simulink model "integrator_ext_IC_test"  (Simulink 8.7)
settings: Solver=ode45  StartTime=0.0  StopTime=10.0  RelTol=1e-3
undefined symbols (not defined in the file or in its folder): DiscIntNeverNeededParam
settings Model: Creator=arnaud  LastModifiedBy=hamza
settings DataIOCC: SaveFormat=Structure  SignalLoggingSaveFormat=ModelDataLogs
settings OptimizationCC: ExpressionDepthLimit=2147483647
settings DebuggingCC: SolverPrmCheckMsg=warning  FcnCallInpInsideContextMsg=UseLocalSettings  StateNameClashWarn=warning
settings GRTTargetCC: CombineOutputUpdateFcns=off  GRTInterface=on
settings ConfigComp: CovSFcnEnable=off

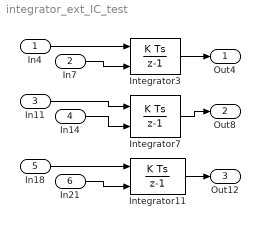
== system integrator_ext_IC_test ==
  In4 : Inport  OutDataTypeStr=double
  In7 : Inport  Port=2  OutDataTypeStr=double
  In11 : Inport  Port=3  OutDataTypeStr=int32
  In14 : Inport  Port=4  OutDataTypeStr=int32
  In18 : Inport  Port=5  OutDataTypeStr=int32
  In21 : Inport  Port=6  OutDataTypeStr=int32
  Integrator11 : DiscreteIntegrator  InitialConditionSource=external  SampleTime=1.0  ICPrevOutput=DiscIntNeverNeededParam  ICPrevScaledInput=DiscIntNeverNeededParam  mask(DiscretizedDiscreteIntegrator){}
      mask init:
      | %zoh
  Integrator3 : DiscreteIntegrator  InitialConditionSource=external  SampleTime=1.0  ICPrevOutput=DiscIntNeverNeededParam  ICPrevScaledInput=DiscIntNeverNeededParam  mask(DiscretizedDiscreteIntegrator){}
      mask init:
      | %zoh
  Integrator7 : DiscreteIntegrator  InitialConditionSource=external  SampleTime=1.0  ICPrevOutput=DiscIntNeverNeededParam  ICPrevScaledInput=DiscIntNeverNeededParam  mask(DiscretizedDiscreteIntegrator){}
      mask init:
      | %zoh
  Out4 : Outport
  Out8 : Outport  Port=2
  Out12 : Outport  Port=3
  wires:
  In4/1 -> Integrator3/1
  Integrator3/1 -> Out4/1
  In7/1 -> Integrator3/2
  In11/1 -> Integrator7/1
  Integrator7/1 -> Out8/1
  In14/1 -> Integrator7/2
  In18/1 -> Integrator11/1
  Integrator11/1 -> Out12/1
  In21/1 -> Integrator11/2
